simulink model "Furuta_sim"  (R2025b)
settings: Solver=FixedStepAuto  StartTime=0.0  StopTime=20  FixedStep=0.00001  RelTol=1e-3
settings Model: Creator=saul-  LastModifiedBy=saul-

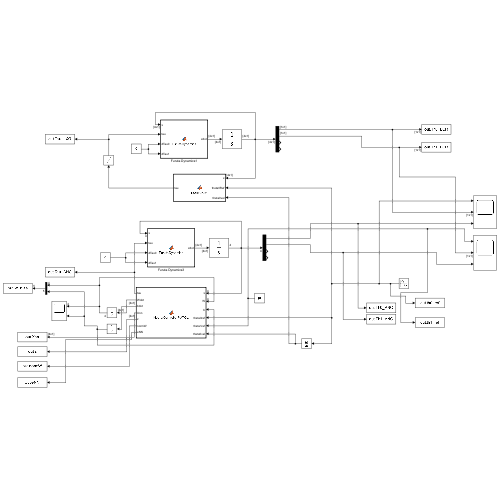
[thumbnail: Simulink's stored preview of the top-level diagram]
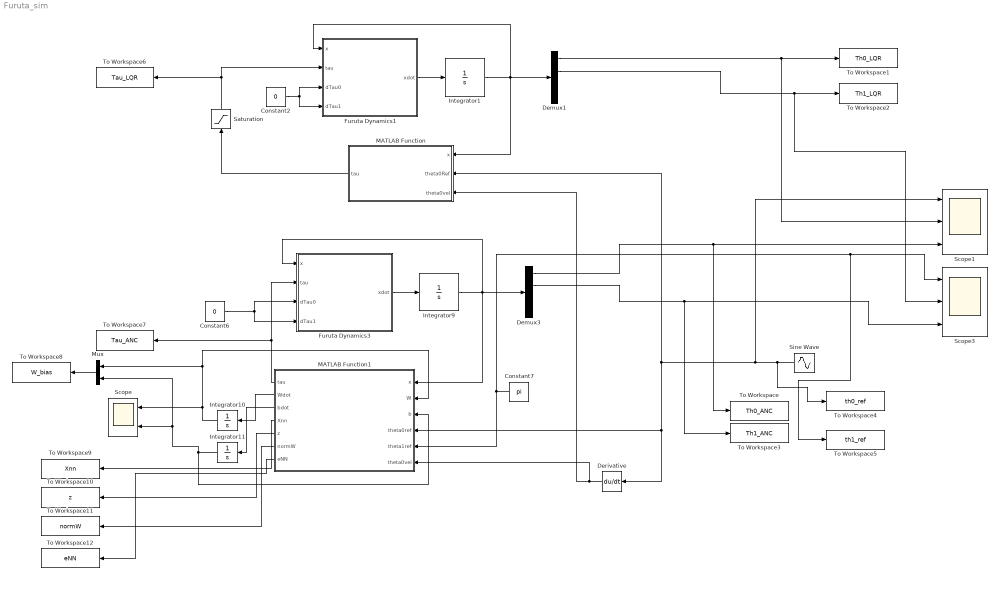
== system Furuta_sim ==
  Constant2 : Constant  Value=0
  Constant6 : Constant  Value=0
  Constant7 : Constant  Value=pi
  Demux1 : Demux
  Demux3 : Demux
  Derivative : Derivative
  Furuta Dynamics1 : MATLAB Function  TreatAsAtomicUnit=on
  Furuta Dynamics3 : MATLAB Function  TreatAsAtomicUnit=on
  Integrator1 : Integrator  InitialCondition=[0;pi;0;0]
  Integrator10 : Integrator  InitialCondition=zeros(4,1)
  Integrator11 : Integrator
  Integrator9 : Integrator  InitialCondition=[0;pi;0;0]
  MATLAB Function : MATLAB Function  TreatAsAtomicUnit=on
  MATLAB Function1 : MATLAB Function  TreatAsAtomicUnit=on
  Mux : Mux  Inputs=2
  Saturation : Saturate  UpperLimit=1  LowerLimit=-1
  Scope : Scope  NumInputPorts=2
      settings: ActiveDisplayYMinimum=-1  ActiveDisplayYMaximum=1
  Scope1 : Scope  NumInputPorts=3
      settings: ActiveDisplayYMinimum=-0.14923366132217819  ActiveDisplayYMaximum=0.14923296562636573
  Scope3 : Scope  NumInputPorts=3
      settings: ActiveDisplayYMinimum=3.1322291369988293  ActiveDisplayYMaximum=3.1454114956497317  DataLoggingVariableName=ScopeData2
  Sine Wave : Sin  Amplitude=0.1  SampleTime=0
  To Workspace : ToWorkspace  VariableName=Th0_ANC  SaveFormat=Timeseries  SampleTime=-1
  To Workspace1 : ToWorkspace  VariableName=Th0_LQR  SaveFormat=Timeseries  SampleTime=-1
  To Workspace10 : ToWorkspace  VariableName=z  SaveFormat=Timeseries  SampleTime=-1
  To Workspace11 : ToWorkspace  VariableName=normW  SaveFormat=Timeseries  SampleTime=-1
  To Workspace12 : ToWorkspace  VariableName=eNN  SaveFormat=Timeseries  SampleTime=-1
  To Workspace2 : ToWorkspace  VariableName=Th1_LQR  SaveFormat=Timeseries  SampleTime=-1
  To Workspace3 : ToWorkspace  VariableName=Th1_ANC  SaveFormat=Timeseries  SampleTime=-1
  To Workspace4 : ToWorkspace  VariableName=th0_ref  SaveFormat=Timeseries  SampleTime=-1
  To Workspace5 : ToWorkspace  VariableName=th1_ref  SaveFormat=Timeseries  SampleTime=-1
  To Workspace6 : ToWorkspace  VariableName=Tau_LQR  SaveFormat=Timeseries  SampleTime=-1
  To Workspace7 : ToWorkspace  VariableName=Tau_ANC  SaveFormat=Timeseries  SampleTime=-1
  To Workspace8 : ToWorkspace  VariableName=W_bias  SaveFormat=Timeseries  SampleTime=-1
  To Workspace9 : ToWorkspace  VariableName=Xnn  SaveFormat=Timeseries  SampleTime=-1
  wires:
  Sine Wave/1 -> To Workspace4/1, MATLAB Function/2(theta0Ref), Derivative/1, MATLAB Function1/4(theta0ref), Scope1/1
  Furuta Dynamics1/1(xdot) -> Integrator1/1
  Integrator1/1 -> MATLAB Function/1(x), Furuta Dynamics1/1(x), Demux1/1
  Constant2/1 -> Furuta Dynamics1/3(dTau0), Furuta Dynamics1/4(dTau1)
  MATLAB Function/1(tau) -> Saturation/1
  Demux1/2 -> Scope3/2, To Workspace2/1
  Demux1/1 -> Scope1/2, To Workspace1/1
  Saturation/1 -> To Workspace6/1, Furuta Dynamics1/2(tau)
  Derivative/1 -> MATLAB Function/3(theta0vel), MATLAB Function1/6(theta0vel)
  Furuta Dynamics3/1(xdot) -> Integrator9/1
  Integrator9/1 -> MATLAB Function1/1(x), Furuta Dynamics3/1(x), Demux3/1
  Constant6/1 -> Furuta Dynamics3/3(dTau0), Furuta Dynamics3/4(dTau1)
  MATLAB Function1/1(tau) -> Furuta Dynamics3/2(tau), To Workspace7/1
  MATLAB Function1/2(Wdot) -> Integrator10/1
  MATLAB Function1/3(bdot) -> Integrator11/1
  Integrator10/1 -> Mux/1, MATLAB Function1/2(W), Scope/1
  Integrator11/1 -> MATLAB Function1/3(b), Mux/2, Scope/2
  Constant7/1 -> To Workspace5/1, Scope3/1, MATLAB Function1/5(theta1ref)
  Demux3/2 -> To Workspace3/1, Scope3/3
  Demux3/1 -> To Workspace/1, Scope1/3
  Mux/1 -> To Workspace8/1
  MATLAB Function1/4(Xnn) -> To Workspace9/1
  MATLAB Function1/5(z) -> To Workspace10/1
  MATLAB Function1/6(normW) -> To Workspace11/1
  MATLAB Function1/7(eNN) -> To Workspace12/1

== matlab function Furuta_sim/Furuta Dynamics1 ==
  data: x input; xdot output; tau input; dTau0 input; dTau1 input
function xdot = FurutaDynamics(x, tau, dTau0, dTau1)
%#codegen
% Dinamica no lineal del pendulo de Furuta
%
% Estado:
%   x(1) = theta0      [rad]   angulo del brazo actuado
%   x(2) = theta1      [rad]   angulo del pendulo
%   x(3) = theta0_dot  [rad/s]
%   x(4) = theta1_dot  [rad/s]
%
% Entrada:
%   tau   = torque del motor [N m]
%   dTau0 = perturbacion externa en eje actuado [N m]
%   dTau1 = perturbacion externa en pivote del pendulo [N m]
%
% Parametros:
%   p = [l0; l1; m1; J0; b0; b1; Fc0; Fc1; epsC; g]

% -----------------------------
% Estados
% -----------------------------
theta0  = x(1);
theta1  = x(2);
theta0d = x(3);
theta1d = x(4);

% -----------------------------
% Parametros
% -----------------------------
l0   = 0.15;        % m
l1   = 0.20;        % m
m1   = 0.05;        % kg
J0   = 1.5e-4;      % kg m^2
b0   = 1.0e-4;      % N m s/rad
b1   = 2.8e-5;      % N m s/rad
Fc0  = 1.5e-3;      % N m
Fc1  = 5.0e-5;      % N m
epsC = 0.01;        % rad/s
g    = 9.81;        % m/s^2

p = [l0; l1; m1; J0; b0; b1; Fc0; Fc1; epsC; g];

l0   = p(1);
l1   = p(2);
m1   = p(3);
J0   = p(4);
b0   = p(5);
b1   = p(6);
Fc0  = p(7);
Fc1  = p(8);
epsC = p(9);
g    = p(10);

lc1 = l1/2;
J1c = (1/12)*m1*l1^2;

% -----------------------------
% Matriz de inercia M(q)
% -----------------------------
M11 = J0 + J1c*sin(theta1)^2 + m1*(l0^2 + lc1^2*sin(theta1)^2);
M12 = m1*l0*lc1*cos(theta1);
M21 = M12;
M22 = J1c + m1*lc1^2;

M = [M11, M12;
     M21, M22];

% -----------------------------
% Terminos centripetos/Coriolis C(q,dq)dq
% -----------------------------
C1 = theta1d*( ...
     2*J1c*theta0d*cos(theta1) ...
   + 2*theta0d*lc1^2*m1*cos(theta1) ...
   - theta1d*l0*lc1*m1) * sin(theta1);

C2 = -0.5*theta0d^2*(J1c + lc1^2*m1)*sin(2*theta1);

Cqd = [C1;
       C2];

% -----------------------------
% Gravedad G(q)
% -----------------------------
G = [0;
     g*lc1*m1*sin(theta1)];

% -----------------------------
% Fuerzas generalizadas Q
% -----------------------------
Q0 = tau + dTau0 ...
     - b0*theta0d ...
     - Fc0*tanh(theta0d/epsC);

Q1 = dTau1 ...
     - b1*theta1d ...
     - Fc1*tanh(theta1d/epsC);

Q = [Q0;
     Q1];

% -----------------------------
% Aceleraciones
% -----------------------------
qdd = M \ (Q - Cqd - G);

theta0dd = qdd(1);
theta1dd = qdd(2);

% -----------------------------
% Salida del sistema
% -----------------------------
xdot = [theta0d;
        theta1d;
        theta0dd;
        theta1dd];
end

== matlab function Furuta_sim/MATLAB Function ==
  data: x input; tau output; theta0Ref input; theta0vel input
function tau = LQRFuruta(x,theta0Ref,theta0vel)
%#codegen
% Control LQR para pendulo de Furuta alrededor de theta1 = pi.
%
% Entrada:
%   x = [theta0; theta1; theta0_dot; theta1_dot]
%
% Salida:
%   tau = torque de control

% Referencias / equilibrio

theta1Eq  = pi;

% Ganancia LQR calculada con el modelo nominal linealizado.
% tau = -K*xerr
K = [-1.0000, 13.6582, -0.717827, 1.68138];

% Vector de error respecto al equilibrio invertido
xerr = zeros(4,1);

xerr(1) = x(1) - theta0Ref;
xerr(2) = x(2) - theta1Eq;
xerr(3) = x(3) - theta0vel;
xerr(4) = x(4);

% Ley LQR
tau = -K*xerr;

end

== matlab function Furuta_sim/MATLAB Function1 ==
  data: x input; tau output; W input; b input; Wdot output; bdot output; theta0ref input; theta1ref input; theta0vel input; Xnn output; z output; normW output; eNN output
function [tau, Wdot, bdot, Xnn, z, normW,eNN] = NeuralControllerPVTOL(x, W, b, theta0ref,theta1ref,theta0vel)

% Control neuronal adaptativo tipo PVTOL para pendulo de Furuta.
%
% Entradas:
%   x = [theta0; theta1; theta0_dot; theta1_dot]
%   W = [w0; w1; w2; w3]
%   b = bias neuronal
%
% Salidas:
%   tau  = torque aplicado al Furuta
%   Wdot = derivada de pesos
%   bdot = derivada del bias
%   eNN  = error ponderado de aprendizaje
%   u    = salida normalizada de la neurona
%   Xnn  = estado normalizado
%   z    = argumento de tanh

% ============================================================
% Referencias
% ============================================================



theta0  = x(1);
theta1  = x(2);
theta0d = x(3);
theta1d = x(4);

Xnn = zeros(4,1);

Xnn(1) = theta0 - theta0ref;
Xnn(2) = theta1 - theta1ref;
Xnn(3) = theta0d - theta0vel;
Xnn(4) = theta1d;

% ============================================================
% Neurona
% ============================================================

z = W.'*Xnn + b;
u = 1*tanh(z);

normW=norm(W);
tau =u;

% ============================================================
% Error ponderado tipo PVTOL
% ============================================================
% En el articulo PVTOL se usa:
%   e = -E X
%
% Para Furuta, elegimos E heuristico.
% Signos elegidos para que el aprendizaje tienda a generar:
%   tau positivo si alpha = theta1 - pi es negativo
%   tau negativo si alpha es positivo
%
% Puedes ajustar estos pesos manualmente.

E = [-0.2;2;-0.2;0.3];

eNN = -(E.'*Xnn);

% ============================================================
% Ley de aprendizaje tipo PVTOL
% ============================================================
% Version continua de:
%   W = W + alpha e X'
%   B = B + alpha e

alpha = 1000;

Wdot = alpha*eNN*Xnn;
bdot = alpha*eNN;

end

== matlab function Furuta_sim/Furuta Dynamics3 ==
  data: x input; xdot output; tau input; dTau0 input; dTau1 input
function xdot = FurutaDynamics(x, tau, dTau0, dTau1)
%#codegen
% Dinamica no lineal del pendulo de Furuta
%
% Estado:
%   x(1) = theta0      [rad]   angulo del brazo actuado
%   x(2) = theta1      [rad]   angulo del pendulo
%   x(3) = theta0_dot  [rad/s]
%   x(4) = theta1_dot  [rad/s]
%
% Entrada:
%   tau   = torque del motor [N m]
%   dTau0 = perturbacion externa en eje actuado [N m]
%   dTau1 = perturbacion externa en pivote del pendulo [N m]
%
% Parametros:
%   p = [l0; l1; m1; J0; b0; b1; Fc0; Fc1; epsC; g]

% -----------------------------
% Estados
% -----------------------------
theta0  = x(1);
theta1  = x(2);
theta0d = x(3);
theta1d = x(4);

% -----------------------------
% Parametros
% -----------------------------
l0   = 0.15;        % m
l1   = 0.20;        % m
m1   = 0.05;        % kg
J0   = 1.5e-4;      % kg m^2
b0   = 1.0e-4;      % N m s/rad
b1   = 2.8e-5;      % N m s/rad
Fc0  = 1.5e-3;      % N m
Fc1  = 5.0e-5;      % N m
epsC = 0.01;        % rad/s
g    = 9.81;        % m/s^2

p = [l0; l1; m1; J0; b0; b1; Fc0; Fc1; epsC; g];

l0   = p(1);
l1   = p(2);
m1   = p(3);
J0   = p(4);
b0   = p(5);
b1   = p(6);
Fc0  = p(7);
Fc1  = p(8);
epsC = p(9);
g    = p(10);

lc1 = l1/2;
J1c = (1/12)*m1*l1^2;

% -----------------------------
% Matriz de inercia M(q)
% -----------------------------
M11 = J0 + J1c*sin(theta1)^2 + m1*(l0^2 + lc1^2*sin(theta1)^2);
M12 = m1*l0*lc1*cos(theta1);
M21 = M12;
M22 = J1c + m1*lc1^2;

M = [M11, M12;
     M21, M22];

% -----------------------------
% Terminos centripetos/Coriolis C(q,dq)dq
% -----------------------------
C1 = theta1d*( ...
     2*J1c*theta0d*cos(theta1) ...
   + 2*theta0d*lc1^2*m1*cos(theta1) ...
   - theta1d*l0*lc1*m1) * sin(theta1);

C2 = -0.5*theta0d^2*(J1c + lc1^2*m1)*sin(2*theta1);

Cqd = [C1;
       C2];

% -----------------------------
% Gravedad G(q)
% -----------------------------
G = [0;
     g*lc1*m1*sin(theta1)];

% -----------------------------
% Fuerzas generalizadas Q
% -----------------------------
Q0 = tau + dTau0 ...
     - b0*theta0d ...
     - Fc0*tanh(theta0d/epsC);

Q1 = dTau1 ...
     - b1*theta1d ...
     - Fc1*tanh(theta1d/epsC);

Q = [Q0;
     Q1];

% -----------------------------
% Aceleraciones
% -----------------------------
qdd = M \ (Q - Cqd - G);

theta0dd = qdd(1);
theta1dd = qdd(2);

% -----------------------------
% Salida del sistema
% -----------------------------
xdot = [theta0d;
        theta1d;
        theta0dd;
        theta1dd];
end
